simulink library "cartToSphere_ul"  (R2022a)
settings: Solver=VariableStepAuto  StartTime=0.0  StopTime=10.0  RelTol=1e-3
settings Model: Creator=jldanie5  LastModifiedBy=lhill8
settings SolverCC: AlgebraicLoopSolver=TrustRegion
settings DebuggingCC: UnconnectedInputMsg=warning  UnconnectedOutputMsg=warning  UnconnectedLineMsg=warning  SFMachineParentedDataDiag=warning  ArithmeticOperatorsInVariantConditions=warning
settings SFSimCC: CustomCodeUndefinedFunction=UseInterfaceOnly

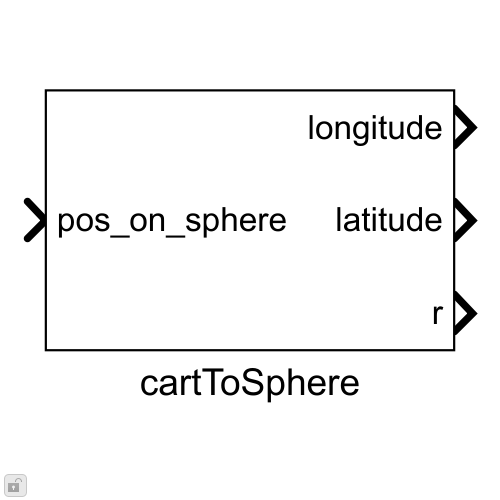
[thumbnail: Simulink's stored preview of the top-level diagram]
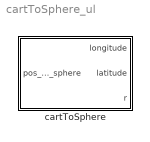
== system cartToSphere_ul ==
  cartToSphere : Subsystem

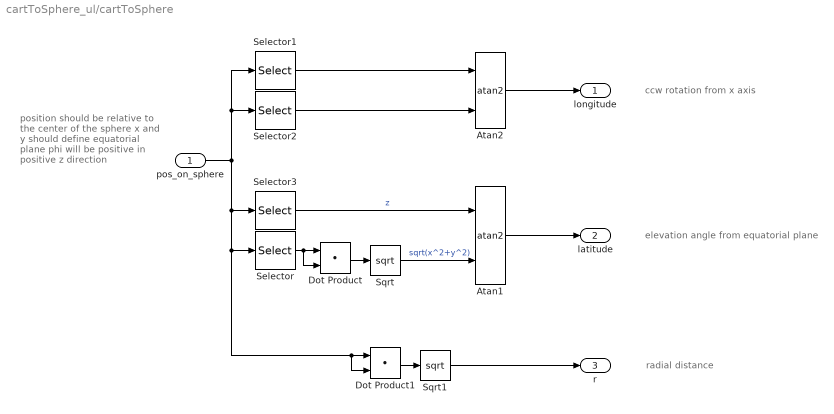
== system cartToSphere_ul/cartToSphere ==
  note: elevation angle from equatorial plane
  note: position should be relative
      | to the center of the sphere
      |
      | x and y should define
      | equatorial plane
      |
      | phi will be positive in
      | positive z direction
  note: ccw rotation from x axis
  note: radial distance
  pos_on_sphere : Inport
  Atan1 : Trigonometry  Operator=atan2
  Atan2 : Trigonometry  Operator=atan2
  Dot Product : DotProduct  OutDataTypeStr=Inherit: Inherit via internal rule
  Dot Product1 : DotProduct  OutDataTypeStr=Inherit: Inherit via internal rule
  Selector : Selector  InputPortWidth=3  IndexOptions=Index vector (dialog)  Indices=[1 2]  OutputSizes=1
  Selector1 : Selector  InputPortWidth=3  IndexOptions=Index vector (dialog)  Indices=2  OutputSizes=1
  Selector2 : Selector  InputPortWidth=3  IndexOptions=Index vector (dialog)  Indices=1  OutputSizes=1
  Selector3 : Selector  InputPortWidth=3  IndexOptions=Index vector (dialog)  Indices=3  OutputSizes=1
  Sqrt : Sqrt
  Sqrt1 : Sqrt
  longitude : Outport  VectorParamsAs1DForOutWhenUnconnected=off
  latitude : Outport  Port=2  VectorParamsAs1DForOutWhenUnconnected=off
  r : Outport  Port=3  VectorParamsAs1DForOutWhenUnconnected=off
  wires:
  Sqrt1/1 -> r/1
  pos_on_sphere/1 -> Selector3/1, Dot Product1/2, Dot Product1/1, Selector/1, Selector1/1, Selector2/1
  Atan2/1 -> longitude/1
  Selector/1 -> Dot Product/2, Dot Product/1
  Dot Product/1 -> Sqrt/1
  Selector3/1 -> Atan1/1  "z"
  Sqrt/1 -> Atan1/2  "sqrt(x^2+y^2)"
  Selector2/1 -> Atan2/2
  Selector1/1 -> Atan2/1
  Atan1/1 -> latitude/1
  Dot Product1/1 -> Sqrt1/1
